simulink model "complex_dbe_core"  (Simulink 7.1)
settings: Solver=ode45  StartTime=0.0  StopTime=1000  RelTol=1e-3
libraries: xbsIndex_r4 x308, cfa_library x64, casper_library_misc x6, simulink x2
(part 3 of 6)

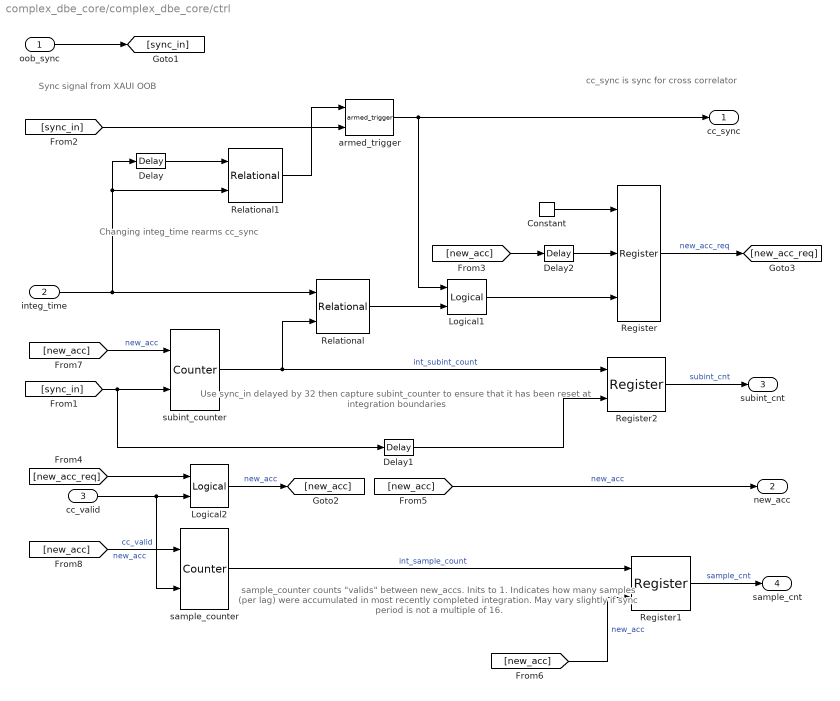
== system complex_dbe_core/complex_dbe_core/ctrl ==
  note: Sync signal from XAUI OOB
  note: cc_sync is sync for
      | cross correlator
  note: Changing integ_time
      | rearms cc_sync
  note: Use sync_in delayed by 32 then capture subint_counter to
      | ensure that it has been reset at integration boundaries
  note: sample_counter counts "valids" between new_accs.  Inits to 1.
      | Indicates how many samples (per lag) were accumulated
      | in most recently completed integration.  May vary slightly if
      | sync period is not a multiple of 16.
  oob_sync : Inport
  integ_time : Inport  Port=2
  cc_valid : Inport  Port=3
  Constant : xbsIndex_r4/Constant  arith_type=Boolean  const=1  n_bits=16  bin_pt=14  explicit_period=on  period=1  equ=P=C  opselect=C  inp2=PCIN>>17  opr=+  inp1=P  carry=CIN  dbl_ovrd=off  block_type=constant
  Delay : xbsIndex_r4/Delay  en=off  latency=1  dbl_ovrd=off  reg_retiming=off  block_type=delay
  Delay1 : xbsIndex_r4/Delay  en=off  latency=32  dbl_ovrd=off  reg_retiming=off  block_type=delay
  Delay2 : xbsIndex_r4/Delay  en=off  latency=2  dbl_ovrd=off  reg_retiming=off  block_type=delay
  Logical1 : xbsIndex_r4/Logical  logical_function=OR  inputs=2  en=off  latency=0  precision=Full  arith_type=Unsigned  n_bits=16  bin_pt=0  align_bp=on  dbl_ovrd=off  block_type=logical
  Logical2 : xbsIndex_r4/Logical  logical_function=AND  inputs=2  en=off  latency=0  precision=Full  arith_type=Unsigned  n_bits=16  bin_pt=0  align_bp=on  dbl_ovrd=off  block_type=logical
  Register : xbsIndex_r4/Register  init=0  rst=on  en=on  dbl_ovrd=off  block_type=register
  Register1 : xbsIndex_r4/Register  init=0  rst=off  en=on  dbl_ovrd=off  block_type=register
  Register2 : xbsIndex_r4/Register  init=0  rst=off  en=on  dbl_ovrd=off  block_type=register
  Relational : xbsIndex_r4/Relational  mode=a=b  en=off  latency=1  dbl_ovrd=off  block_type=relational
      settings: block_version=10.1.3
  Relational1 : xbsIndex_r4/Relational  mode=a=b  en=off  latency=1  dbl_ovrd=off  block_type=relational
      settings: block_version=10.1.3
  armed_trigger : casper_library_misc/armed_trigger  SystemSampleTime=-1  hidden=0
  sample_counter : xbsIndex_r4/Counter  cnt_type=Free Running  cnt_to=Inf  operation=Up  start_count=1  cnt_by_val=1  arith_type=Unsigned  n_bits=32  bin_pt=0  load_pin=off  rst=on  en=on  explicit_period=on  period=1  dbl_ovrd=off  use_behavioral_HDL=off  use_rpm=off  implementation=Fabric  block_type=counter
  subint_counter : xbsIndex_r4/Counter  cnt_type=Free Running  cnt_to=Inf  operation=Up  start_count=0  cnt_by_val=1  arith_type=Unsigned  n_bits=32  bin_pt=0  load_pin=off  rst=on  en=on  explicit_period=on  period=1  dbl_ovrd=off  use_behavioral_HDL=off  use_rpm=off  implementation=Fabric  block_type=counter
  cc_sync : Outport
  new_acc : Outport  Port=2
  subint_cnt : Outport  Port=3
  sample_cnt : Outport  Port=4
  wires:
  armed_trigger/1 -> cc_sync/1, Logical1/1
  oob_sync/1 -> [sync_in]
  [new_acc] -> subint_counter/1  "new_acc"
  [sync_in] -> subint_counter/2, Delay1/1
  integ_time/1 -> Delay/1, Relational1/2, Relational/1
  Relational/1 -> Logical1/2
  Logical1/1 -> Register/3
  Delay/1 -> Relational1/1
  subint_counter/1 -> Relational/2, Register2/1  "int_subint_count"
  Relational1/1 -> armed_trigger/1
  [sync_in] -> armed_trigger/2
  Register/1 -> [new_acc_req]  "new_acc_req"
  [new_acc] -> Delay2/1
  Constant/1 -> Register/1
  Delay2/1 -> Register/2
  Delay1/1 -> Register2/2
  Register2/1 -> subint_cnt/1  "subint_cnt"
  [new_acc_req] -> Logical2/1
  cc_valid/1 -> Logical2/2, sample_counter/2  "cc_valid"
  Logical2/1 -> [new_acc]  "new_acc"
  [new_acc] -> new_acc/1  "new_acc"
  [new_acc] -> sample_counter/1  "new_acc"
  sample_counter/1 -> Register1/1  "int_sample_count"
  [new_acc] -> Register1/2  "new_acc"
  Register1/1 -> sample_cnt/1  "sample_cnt"

== system complex_dbe_core/complex_dbe_core/edge_detect ==
  in : Inport  OutDataType=sfix(16)  OutScaling=2^0
  Delay : xbsIndex_r4/Delay  en=off  latency=1  dbl_ovrd=off  reg_retiming=off  block_type=delay
      settings: xl_area=[0, 0, 0, 0, 0, 0, 0]
  Inverter : xbsIndex_r4/Inverter  en=off  latency=0  dbl_ovrd=off  block_type=inv
      settings: xl_area=[0, 0, 0, 0, 0, 0, 0]
  edge_op : xbsIndex_r4/Logical  logical_function=AND  inputs=2  en=off  latency=0  precision=Full  arith_type=Unsigned  n_bits=8  bin_pt=2  align_bp=on  dbl_ovrd=off  block_type=logical
      settings: xl_area=[0, 0, 0, 0, 0, 0, 0]
  out : Outport  OutDataType=sfix(16)  OutScaling=2^0
  wires:
  Inverter/1 -> edge_op/1
  edge_op/1 -> out/1
  in/1 -> Inverter/1, Delay/1
  Delay/1 -> edge_op/2

== system complex_dbe_core/complex_dbe_core/edge_detect1 ==
  in : Inport  OutDataType=sfix(16)  OutScaling=2^0
  Delay : xbsIndex_r4/Delay  en=off  latency=1  dbl_ovrd=off  reg_retiming=off  block_type=delay
      settings: xl_area=[0, 0, 0, 0, 0, 0, 0]
  Inverter : xbsIndex_r4/Inverter  en=off  latency=0  dbl_ovrd=off  block_type=inv
      settings: xl_area=[0, 0, 0, 0, 0, 0, 0]
  edge_op : xbsIndex_r4/Logical  logical_function=AND  inputs=2  en=off  latency=0  precision=Full  arith_type=Unsigned  n_bits=8  bin_pt=2  align_bp=on  dbl_ovrd=off  block_type=logical
      settings: xl_area=[0, 0, 0, 0, 0, 0, 0]
  out : Outport  OutDataType=sfix(16)  OutScaling=2^0
  wires:
  Inverter/1 -> edge_op/1
  edge_op/1 -> out/1
  in/1 -> Inverter/1, Delay/1
  Delay/1 -> edge_op/2

== system complex_dbe_core/complex_dbe_core/usb_imag_bram_vacc ==
  new_acc : Inport
  din : Inport  Port=2
  Delay1 : xbsIndex_r4/Delay  en=off  latency=1  dbl_ovrd=off  reg_retiming=off  block_type=delay
  Delay2 : xbsIndex_r4/Delay  en=off  latency=1  dbl_ovrd=off  reg_retiming=off  block_type=delay
  Delay5 : xbsIndex_r4/Delay  en=off  latency=2  dbl_ovrd=off  reg_retiming=off  block_type=delay
      settings: block_version=11.4
  Delay6 : xbsIndex_r4/Delay  en=off  latency=2  dbl_ovrd=off  reg_retiming=off  block_type=delay
      settings: block_version=11.4
  Reinterpret : xbsIndex_r4/Reinterpret  force_arith_type=off  arith_type=Unsigned  force_bin_pt=on  bin_pt=4  block_type=reinterpret
      settings: infoedit="Changes signal type without altering the binary representation.   You can changed the signal between signed and unsigned, and relocate the binary point.<P><P>Hardware notes: In hardware this block costs nothing.<P><P>Example:  Suppose the input is 6 bits wide, signed, with 2 fractional bits, and the output is forced to unsigned with 0 fractional bits.  Then an input of -2.0 (1110.00 in binary 2's complement) becomes an output of 56 (111000 in binary)."  block_version=10.1.3
  addr_bram_vacc : Subsystem  AncestorBlock=casper_library_accumulators/addr_bram_vacc  mask(simple_bram_vacc){vec_len=16, arith_type=Signed, n_bits=36, bin_pt=0}
      mask prompts: vec_len "Vector length:"; arith_type "Output type:"; n_bits "Bit width (output):"; bin_pt "Binary point (output):"
      mask help: This simple vector accumulator is based on a shift register. It outputs its previous accumulated vector after a new_acc pulse is received.
      mask init:
      | simple_bram_vacc_init(gcb, ...
      |     'vec_len', vec_len, ...
      |     'arith_type', arith_type, ...
      |     'n_bits', n_bits, ...
      |     'bin_pt', bin_pt);
      mask StyleString: edit,popup(Signed|Unsigned),edit,edit
  convert : Subsystem  AncestorBlock=casper_library_misc/convert  mask(convert){bin_pt_in=4, n_bits_out=32, bin_pt_out=0, quantization=Round  (unbiased: Even Values), overflow=Wrap, latency=1}
      mask prompts: bin_pt_in "Binary Point In"; n_bits_out "Bit Width Out"; bin_pt_out "Binary Point Out"
      mask help:
      | Convert input value to the specified bit width and precision.
      |
      | Does not support upscaling number of fractional bits (eg 8_5 to 8_4 is ok, but not 8_4 to 8_5).
      mask init:
      | convert_init(gcb, ...
      |     'bin_pt_in',bin_pt_in, ...
      |     'n_bits_out',n_bits_out,...
      |     'bin_pt_out',bin_pt_out, ...
      |     'quantization',quantization,...
      |     'overflow',overflow,...
      |     'latency',latency);
      settings: AttributesFormatString=|
      | N_4 ==> 32_0
      | round even, wrap
      | latency = 1
      mask Help:
      | <pre>
      | Description::
      | 
      | Outputs converted version of the input.
      | 
      | Mask Parameters::
      | 
      | Binary Point In (bin_pt_in): Specifies the binary point location in the input.
      | 
      | Bit Width Out (n_bits_out): Specifies the width of the output.
      | 
      | Binary Point Out (bin_pt_out): Specifies the binary point location in the output.
      | 
      | Quantization (quantization): Specifies quantization handling.
      | 
      | Overflow (overflow): Specifies overflow handling.
      | 
      | Latency (latency): Specifies the latency of the underlying adder block, which is the overall
      | latency of this block as well.
      | </pre>
      mask StyleString: edit,edit,edit,popup(Truncate|Round  (unbiased: +/- Inf)|Round  (unbiased: Even Values)|Round  (unbiased: Zero)|Round  (unbiased: Odd Values)|Round  (biased: Up)|Round  (biased: Down)),popup(Wrap|Saturate|Error),edit
  addr : Outport
  dout : Outport  Port=2
  we : Outport  Port=3
  wires:
  Delay5/1 -> addr_bram_vacc/1(new_acc)  "bv_new_acc"
  Delay6/1 -> addr_bram_vacc/2(din)  "bv_din"
  new_acc/1 -> Delay5/1
  addr_bram_vacc/2(dout) -> Reinterpret/1
  din/1 -> Delay6/1
  addr_bram_vacc/3(we) -> Delay2/1
  addr_bram_vacc/1(addr) -> Delay1/1
  Reinterpret/1 -> convert/1(in)
  convert/1(out) -> dout/1
  Delay1/1 -> addr/1
  Delay2/1 -> we/1

== system complex_dbe_core/complex_dbe_core/usb_real_bram_vacc ==
  new_acc : Inport
  din : Inport  Port=2
  Delay1 : xbsIndex_r4/Delay  en=off  latency=1  dbl_ovrd=off  reg_retiming=off  block_type=delay
  Delay2 : xbsIndex_r4/Delay  en=off  latency=1  dbl_ovrd=off  reg_retiming=off  block_type=delay
  Delay5 : xbsIndex_r4/Delay  en=off  latency=2  dbl_ovrd=off  reg_retiming=off  block_type=delay
      settings: block_version=11.4
  Delay6 : xbsIndex_r4/Delay  en=off  latency=2  dbl_ovrd=off  reg_retiming=off  block_type=delay
      settings: block_version=11.4
  Reinterpret : xbsIndex_r4/Reinterpret  force_arith_type=off  arith_type=Unsigned  force_bin_pt=on  bin_pt=4  block_type=reinterpret
      settings: infoedit="Changes signal type without altering the binary representation.   You can changed the signal between signed and unsigned, and relocate the binary point.<P><P>Hardware notes: In hardware this block costs nothing.<P><P>Example:  Suppose the input is 6 bits wide, signed, with 2 fractional bits, and the output is forced to unsigned with 0 fractional bits.  Then an input of -2.0 (1110.00 in binary 2's complement) becomes an output of 56 (111000 in binary)."  block_version=10.1.3
  addr_bram_vacc : Subsystem  AncestorBlock=casper_library_accumulators/addr_bram_vacc  mask(simple_bram_vacc){vec_len=16, arith_type=Signed, n_bits=36, bin_pt=0}
      mask prompts: vec_len "Vector length:"; arith_type "Output type:"; n_bits "Bit width (output):"; bin_pt "Binary point (output):"
      mask help: This simple vector accumulator is based on a shift register. It outputs its previous accumulated vector after a new_acc pulse is received.
      mask init:
      | simple_bram_vacc_init(gcb, ...
      |     'vec_len', vec_len, ...
      |     'arith_type', arith_type, ...
      |     'n_bits', n_bits, ...
      |     'bin_pt', bin_pt);
      mask StyleString: edit,popup(Signed|Unsigned),edit,edit
  convert : Subsystem  AncestorBlock=casper_library_misc/convert  mask(convert){bin_pt_in=4, n_bits_out=32, bin_pt_out=0, quantization=Round  (unbiased: Even Values), overflow=Wrap, latency=1}
      mask prompts: bin_pt_in "Binary Point In"; n_bits_out "Bit Width Out"; bin_pt_out "Binary Point Out"
      mask help:
      | Convert input value to the specified bit width and precision.
      |
      | Does not support upscaling number of fractional bits (eg 8_5 to 8_4 is ok, but not 8_4 to 8_5).
      mask init: same as complex_dbe_core/complex_dbe_core/usb_imag_bram_vacc/convert
      settings: AttributesFormatString=|
      | N_4 ==> 32_0
      | round even, wrap
      | latency = 1
      mask Help:
      | <pre>
      | Description::
      | 
      | Outputs converted version of the input.
      | 
      | Mask Parameters::
      | 
      | Binary Point In (bin_pt_in): Specifies the binary point location in the input.
      | 
      | Bit Width Out (n_bits_out): Specifies the width of the output.
      | 
      | Binary Point Out (bin_pt_out): Specifies the binary point location in the output.
      | 
      | Quantization (quantization): Specifies quantization handling.
      | 
      | Overflow (overflow): Specifies overflow handling.
      | 
      | Latency (latency): Specifies the latency of the underlying adder block, which is the overall
      | latency of this block as well.
      | </pre>
      mask StyleString: edit,edit,edit,popup(Truncate|Round  (unbiased: +/- Inf)|Round  (unbiased: Even Values)|Round  (unbiased: Zero)|Round  (unbiased: Odd Values)|Round  (biased: Up)|Round  (biased: Down)),popup(Wrap|Saturate|Error),edit
  addr : Outport
  dout : Outport  Port=2
  we : Outport  Port=3
  wires:
  Delay5/1 -> addr_bram_vacc/1(new_acc)  "bv_new_acc"
  Delay6/1 -> addr_bram_vacc/2(din)  "bv_din"
  new_acc/1 -> Delay5/1
  addr_bram_vacc/2(dout) -> Reinterpret/1
  din/1 -> Delay6/1
  addr_bram_vacc/3(we) -> Delay2/1
  addr_bram_vacc/1(addr) -> Delay1/1
  Reinterpret/1 -> convert/1(in)
  convert/1(out) -> dout/1
  Delay1/1 -> addr/1
  Delay2/1 -> we/1

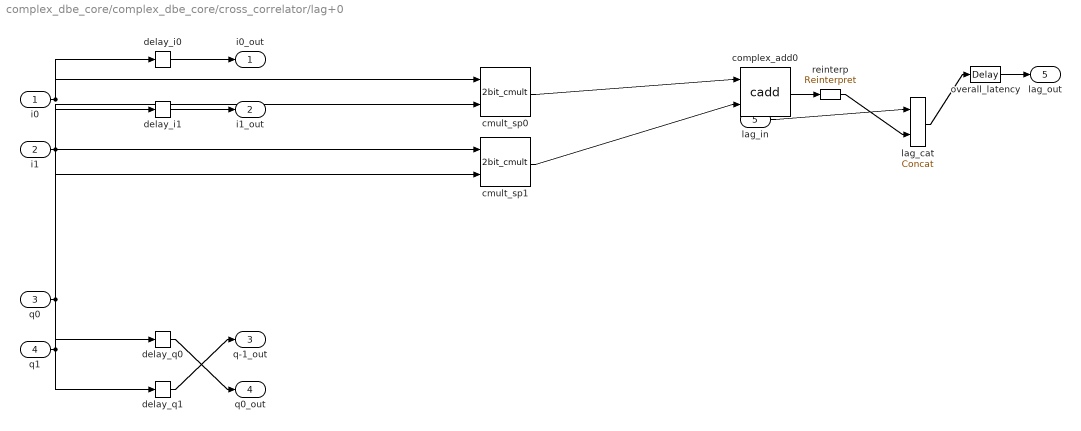
== system complex_dbe_core/complex_dbe_core/cross_correlator/lag+0 ==
  i0 : Inport
  i1 : Inport  Port=2
  q0 : Inport  Port=3
  q1 : Inport  Port=4
  lag_in : Inport  Port=5
  cmult_sp0 : cfa_library/2bit_cmult  SystemSampleTime=-1  add_delay=2
  cmult_sp1 : cfa_library/2bit_cmult  SystemSampleTime=-1  add_delay=2
  complex_add0 : cfa_library/cadd  SystemSampleTime=-1  input_bit_width=6  input_bin_pt=0  add_delay=2
  delay_i0 : xbsIndex_r4/Delay  en=off  latency=2  dbl_ovrd=off  reg_retiming=off  block_type=delay
      settings: block_version=11.4
  delay_i1 : xbsIndex_r4/Delay  en=off  latency=2  dbl_ovrd=off  reg_retiming=off  block_type=delay
      settings: block_version=11.4
  delay_q0 : xbsIndex_r4/Delay  en=off  latency=1  dbl_ovrd=off  reg_retiming=off  block_type=delay
      settings: block_version=11.4
  delay_q1 : xbsIndex_r4/Delay  en=off  latency=2  dbl_ovrd=off  reg_retiming=off  block_type=delay
      settings: block_version=11.4
  lag_cat : xbsIndex_r4/Concat  num_inputs=2  dbl_ovrd=off  block_type=concat
  overall_latency : xbsIndex_r4/Delay  en=off  latency=2  dbl_ovrd=off  reg_retiming=on  block_type=delay
  reinterp : xbsIndex_r4/Reinterpret  force_arith_type=on  arith_type=Unsigned  force_bin_pt=on  bin_pt=0  block_type=reinterpret
      settings: infoedit="Changes signal type without altering the binary representation.   You can changed the signal between signed and unsigned, and relocate the binary point.<br><br>Hardware notes: In hardware this block costs nothing.<br><br>Example:  Suppose the input is 6 bits wide, signed, with 2 fractional bits, and the output is forced to unsigned with 0 fractional bits.  Then an input of -2.0 (1110.00 in binary 2's complement) becomes an output of 56 (111000 in binary)."
  i0_out : Outport
  i1_out : Outport  Port=2
  q-1_out : Outport  Port=3
  q0_out : Outport  Port=4
  lag_out : Outport  Port=5
  wires:
  i0/1 -> cmult_sp0/1, delay_i0/1
  q0/1 -> cmult_sp0/2, delay_q0/1
  i1/1 -> cmult_sp1/1, delay_i1/1
  q1/1 -> cmult_sp1/2, delay_q1/1
  cmult_sp0/1 -> complex_add0/1
  cmult_sp1/1 -> complex_add0/2
  delay_i0/1 -> i0_out/1
  delay_q0/1 -> q0_out/1
  delay_i1/1 -> i1_out/1
  delay_q1/1 -> q-1_out/1
  lag_in/1 -> lag_cat/1
  complex_add0/1 -> reinterp/1
  reinterp/1 -> lag_cat/2
  lag_cat/1 -> overall_latency/1
  overall_latency/1 -> lag_out/1

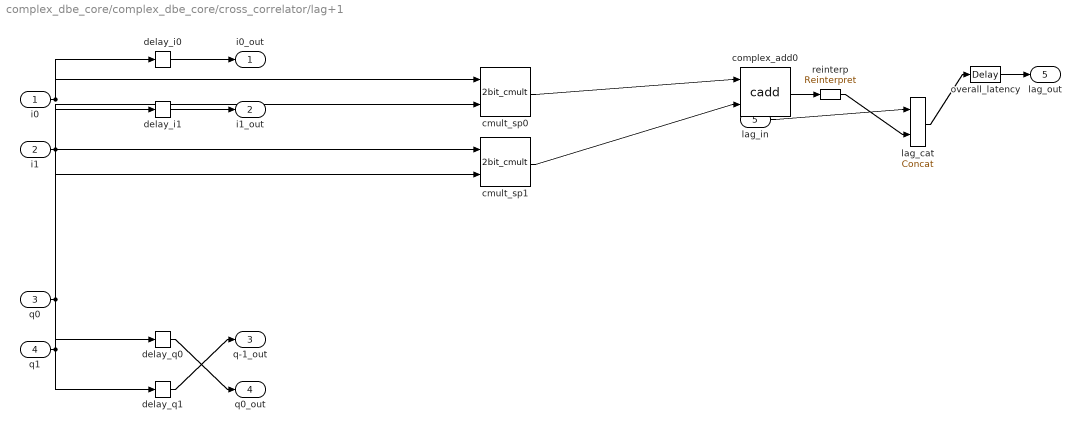
== system complex_dbe_core/complex_dbe_core/cross_correlator/lag+1 ==
  i0 : Inport
  i1 : Inport  Port=2
  q0 : Inport  Port=3
  q1 : Inport  Port=4
  lag_in : Inport  Port=5
  cmult_sp0 : cfa_library/2bit_cmult  SystemSampleTime=-1  add_delay=2
  cmult_sp1 : cfa_library/2bit_cmult  SystemSampleTime=-1  add_delay=2
  complex_add0 : cfa_library/cadd  SystemSampleTime=-1  input_bit_width=6  input_bin_pt=0  add_delay=2
  delay_i0 : xbsIndex_r4/Delay  en=off  latency=2  dbl_ovrd=off  reg_retiming=off  block_type=delay
      settings: block_version=11.4
  delay_i1 : xbsIndex_r4/Delay  en=off  latency=2  dbl_ovrd=off  reg_retiming=off  block_type=delay
      settings: block_version=11.4
  delay_q0 : xbsIndex_r4/Delay  en=off  latency=1  dbl_ovrd=off  reg_retiming=off  block_type=delay
      settings: block_version=11.4
  delay_q1 : xbsIndex_r4/Delay  en=off  latency=2  dbl_ovrd=off  reg_retiming=off  block_type=delay
      settings: block_version=11.4
  lag_cat : xbsIndex_r4/Concat  num_inputs=2  dbl_ovrd=off  block_type=concat
  overall_latency : xbsIndex_r4/Delay  en=off  latency=2  dbl_ovrd=off  reg_retiming=on  block_type=delay
  reinterp : xbsIndex_r4/Reinterpret  force_arith_type=on  arith_type=Unsigned  force_bin_pt=on  bin_pt=0  block_type=reinterpret
      settings: infoedit="Changes signal type without altering the binary representation.   You can changed the signal between signed and unsigned, and relocate the binary point.<br><br>Hardware notes: In hardware this block costs nothing.<br><br>Example:  Suppose the input is 6 bits wide, signed, with 2 fractional bits, and the output is forced to unsigned with 0 fractional bits.  Then an input of -2.0 (1110.00 in binary 2's complement) becomes an output of 56 (111000 in binary)."
  i0_out : Outport
  i1_out : Outport  Port=2
  q-1_out : Outport  Port=3
  q0_out : Outport  Port=4
  lag_out : Outport  Port=5
  wires:
  i0/1 -> cmult_sp0/1, delay_i0/1
  q0/1 -> cmult_sp0/2, delay_q0/1
  i1/1 -> cmult_sp1/1, delay_i1/1
  q1/1 -> cmult_sp1/2, delay_q1/1
  cmult_sp0/1 -> complex_add0/1
  cmult_sp1/1 -> complex_add0/2
  delay_i0/1 -> i0_out/1
  delay_q0/1 -> q0_out/1
  delay_i1/1 -> i1_out/1
  delay_q1/1 -> q-1_out/1
  lag_in/1 -> lag_cat/1
  complex_add0/1 -> reinterp/1
  reinterp/1 -> lag_cat/2
  lag_cat/1 -> overall_latency/1
  overall_latency/1 -> lag_out/1

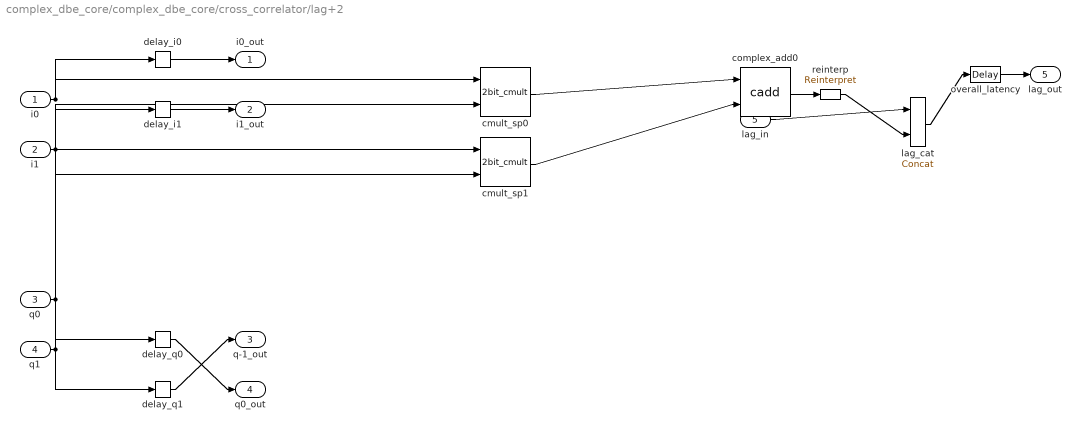
== system complex_dbe_core/complex_dbe_core/cross_correlator/lag+2 ==
  i0 : Inport
  i1 : Inport  Port=2
  q0 : Inport  Port=3
  q1 : Inport  Port=4
  lag_in : Inport  Port=5
  cmult_sp0 : cfa_library/2bit_cmult  SystemSampleTime=-1  add_delay=2
  cmult_sp1 : cfa_library/2bit_cmult  SystemSampleTime=-1  add_delay=2
  complex_add0 : cfa_library/cadd  SystemSampleTime=-1  input_bit_width=6  input_bin_pt=0  add_delay=2
  delay_i0 : xbsIndex_r4/Delay  en=off  latency=2  dbl_ovrd=off  reg_retiming=off  block_type=delay
      settings: block_version=11.4
  delay_i1 : xbsIndex_r4/Delay  en=off  latency=2  dbl_ovrd=off  reg_retiming=off  block_type=delay
      settings: block_version=11.4
  delay_q0 : xbsIndex_r4/Delay  en=off  latency=1  dbl_ovrd=off  reg_retiming=off  block_type=delay
      settings: block_version=11.4
  delay_q1 : xbsIndex_r4/Delay  en=off  latency=2  dbl_ovrd=off  reg_retiming=off  block_type=delay
      settings: block_version=11.4
  lag_cat : xbsIndex_r4/Concat  num_inputs=2  dbl_ovrd=off  block_type=concat
  overall_latency : xbsIndex_r4/Delay  en=off  latency=2  dbl_ovrd=off  reg_retiming=on  block_type=delay
  reinterp : xbsIndex_r4/Reinterpret  force_arith_type=on  arith_type=Unsigned  force_bin_pt=on  bin_pt=0  block_type=reinterpret
      settings: infoedit="Changes signal type without altering the binary representation.   You can changed the signal between signed and unsigned, and relocate the binary point.<br><br>Hardware notes: In hardware this block costs nothing.<br><br>Example:  Suppose the input is 6 bits wide, signed, with 2 fractional bits, and the output is forced to unsigned with 0 fractional bits.  Then an input of -2.0 (1110.00 in binary 2's complement) becomes an output of 56 (111000 in binary)."
  i0_out : Outport
  i1_out : Outport  Port=2
  q-1_out : Outport  Port=3
  q0_out : Outport  Port=4
  lag_out : Outport  Port=5
  wires:
  i0/1 -> cmult_sp0/1, delay_i0/1
  q0/1 -> cmult_sp0/2, delay_q0/1
  i1/1 -> cmult_sp1/1, delay_i1/1
  q1/1 -> cmult_sp1/2, delay_q1/1
  cmult_sp0/1 -> complex_add0/1
  cmult_sp1/1 -> complex_add0/2
  delay_i0/1 -> i0_out/1
  delay_q0/1 -> q0_out/1
  delay_i1/1 -> i1_out/1
  delay_q1/1 -> q-1_out/1
  lag_in/1 -> lag_cat/1
  complex_add0/1 -> reinterp/1
  reinterp/1 -> lag_cat/2
  lag_cat/1 -> overall_latency/1
  overall_latency/1 -> lag_out/1

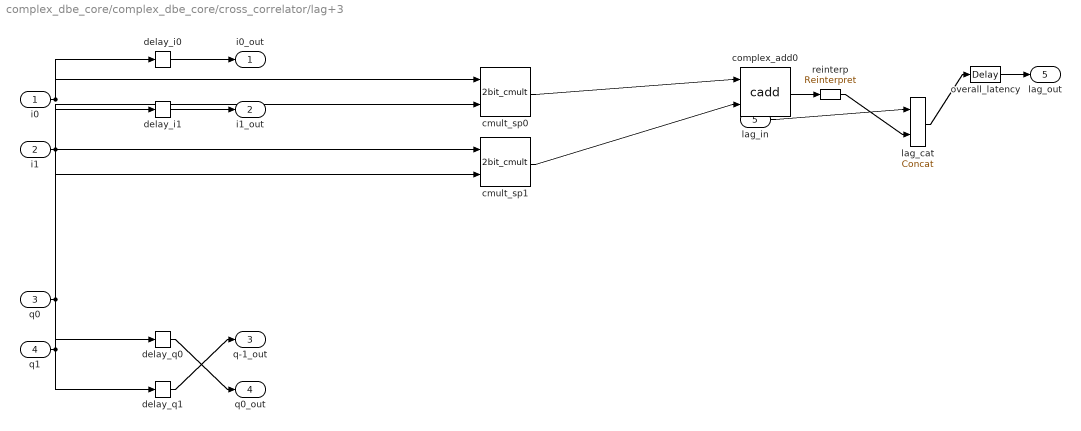
== system complex_dbe_core/complex_dbe_core/cross_correlator/lag+3 ==
  i0 : Inport
  i1 : Inport  Port=2
  q0 : Inport  Port=3
  q1 : Inport  Port=4
  lag_in : Inport  Port=5
  cmult_sp0 : cfa_library/2bit_cmult  SystemSampleTime=-1  add_delay=2
  cmult_sp1 : cfa_library/2bit_cmult  SystemSampleTime=-1  add_delay=2
  complex_add0 : cfa_library/cadd  SystemSampleTime=-1  input_bit_width=6  input_bin_pt=0  add_delay=2
  delay_i0 : xbsIndex_r4/Delay  en=off  latency=2  dbl_ovrd=off  reg_retiming=off  block_type=delay
      settings: block_version=11.4
  delay_i1 : xbsIndex_r4/Delay  en=off  latency=2  dbl_ovrd=off  reg_retiming=off  block_type=delay
      settings: block_version=11.4
  delay_q0 : xbsIndex_r4/Delay  en=off  latency=1  dbl_ovrd=off  reg_retiming=off  block_type=delay
      settings: block_version=11.4
  delay_q1 : xbsIndex_r4/Delay  en=off  latency=2  dbl_ovrd=off  reg_retiming=off  block_type=delay
      settings: block_version=11.4
  lag_cat : xbsIndex_r4/Concat  num_inputs=2  dbl_ovrd=off  block_type=concat
  overall_latency : xbsIndex_r4/Delay  en=off  latency=2  dbl_ovrd=off  reg_retiming=on  block_type=delay
  reinterp : xbsIndex_r4/Reinterpret  force_arith_type=on  arith_type=Unsigned  force_bin_pt=on  bin_pt=0  block_type=reinterpret
      settings: infoedit="Changes signal type without altering the binary representation.   You can changed the signal between signed and unsigned, and relocate the binary point.<br><br>Hardware notes: In hardware this block costs nothing.<br><br>Example:  Suppose the input is 6 bits wide, signed, with 2 fractional bits, and the output is forced to unsigned with 0 fractional bits.  Then an input of -2.0 (1110.00 in binary 2's complement) becomes an output of 56 (111000 in binary)."
  i0_out : Outport
  i1_out : Outport  Port=2
  q-1_out : Outport  Port=3
  q0_out : Outport  Port=4
  lag_out : Outport  Port=5
  wires:
  i0/1 -> cmult_sp0/1, delay_i0/1
  q0/1 -> cmult_sp0/2, delay_q0/1
  i1/1 -> cmult_sp1/1, delay_i1/1
  q1/1 -> cmult_sp1/2, delay_q1/1
  cmult_sp0/1 -> complex_add0/1
  cmult_sp1/1 -> complex_add0/2
  delay_i0/1 -> i0_out/1
  delay_q0/1 -> q0_out/1
  delay_i1/1 -> i1_out/1
  delay_q1/1 -> q-1_out/1
  lag_in/1 -> lag_cat/1
  complex_add0/1 -> reinterp/1
  reinterp/1 -> lag_cat/2
  lag_cat/1 -> overall_latency/1
  overall_latency/1 -> lag_out/1

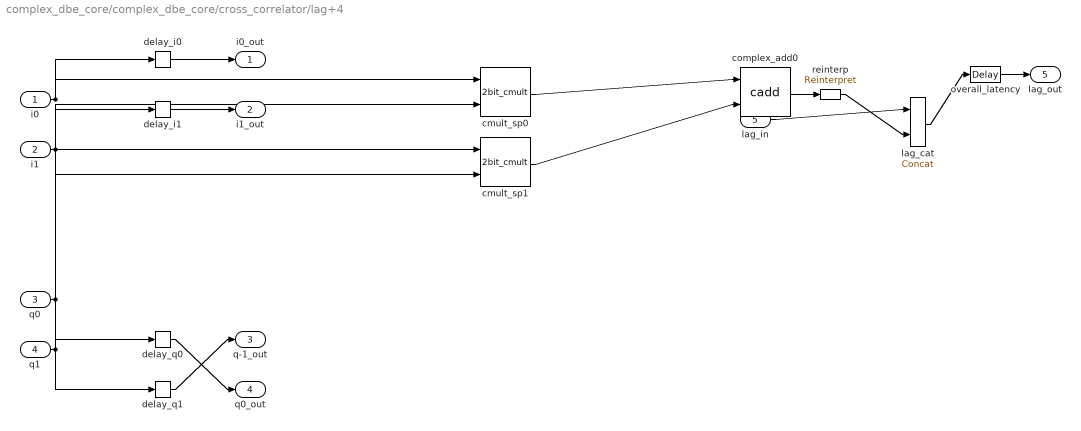
== system complex_dbe_core/complex_dbe_core/cross_correlator/lag+4 ==
  i0 : Inport
  i1 : Inport  Port=2
  q0 : Inport  Port=3
  q1 : Inport  Port=4
  lag_in : Inport  Port=5
  cmult_sp0 : cfa_library/2bit_cmult  SystemSampleTime=-1  add_delay=2
  cmult_sp1 : cfa_library/2bit_cmult  SystemSampleTime=-1  add_delay=2
  complex_add0 : cfa_library/cadd  SystemSampleTime=-1  input_bit_width=6  input_bin_pt=0  add_delay=2
  delay_i0 : xbsIndex_r4/Delay  en=off  latency=2  dbl_ovrd=off  reg_retiming=off  block_type=delay
      settings: block_version=11.4
  delay_i1 : xbsIndex_r4/Delay  en=off  latency=2  dbl_ovrd=off  reg_retiming=off  block_type=delay
      settings: block_version=11.4
  delay_q0 : xbsIndex_r4/Delay  en=off  latency=1  dbl_ovrd=off  reg_retiming=off  block_type=delay
      settings: block_version=11.4
  delay_q1 : xbsIndex_r4/Delay  en=off  latency=2  dbl_ovrd=off  reg_retiming=off  block_type=delay
      settings: block_version=11.4
  lag_cat : xbsIndex_r4/Concat  num_inputs=2  dbl_ovrd=off  block_type=concat
  overall_latency : xbsIndex_r4/Delay  en=off  latency=2  dbl_ovrd=off  reg_retiming=on  block_type=delay
  reinterp : xbsIndex_r4/Reinterpret  force_arith_type=on  arith_type=Unsigned  force_bin_pt=on  bin_pt=0  block_type=reinterpret
      settings: infoedit="Changes signal type without altering the binary representation.   You can changed the signal between signed and unsigned, and relocate the binary point.<br><br>Hardware notes: In hardware this block costs nothing.<br><br>Example:  Suppose the input is 6 bits wide, signed, with 2 fractional bits, and the output is forced to unsigned with 0 fractional bits.  Then an input of -2.0 (1110.00 in binary 2's complement) becomes an output of 56 (111000 in binary)."
  i0_out : Outport
  i1_out : Outport  Port=2
  q-1_out : Outport  Port=3
  q0_out : Outport  Port=4
  lag_out : Outport  Port=5
  wires:
  i0/1 -> cmult_sp0/1, delay_i0/1
  q0/1 -> cmult_sp0/2, delay_q0/1
  i1/1 -> cmult_sp1/1, delay_i1/1
  q1/1 -> cmult_sp1/2, delay_q1/1
  cmult_sp0/1 -> complex_add0/1
  cmult_sp1/1 -> complex_add0/2
  delay_i0/1 -> i0_out/1
  delay_q0/1 -> q0_out/1
  delay_i1/1 -> i1_out/1
  delay_q1/1 -> q-1_out/1
  lag_in/1 -> lag_cat/1
  complex_add0/1 -> reinterp/1
  reinterp/1 -> lag_cat/2
  lag_cat/1 -> overall_latency/1
  overall_latency/1 -> lag_out/1

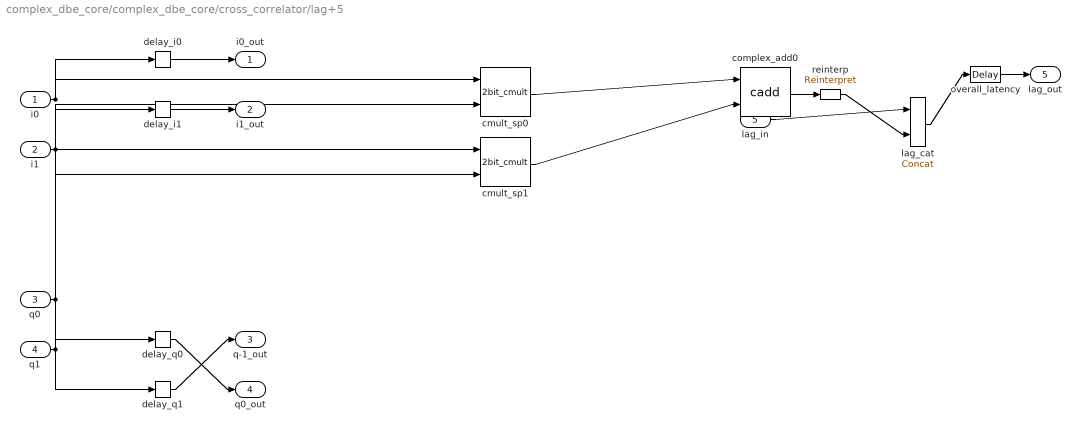
== system complex_dbe_core/complex_dbe_core/cross_correlator/lag+5 ==
  i0 : Inport
  i1 : Inport  Port=2
  q0 : Inport  Port=3
  q1 : Inport  Port=4
  lag_in : Inport  Port=5
  cmult_sp0 : cfa_library/2bit_cmult  SystemSampleTime=-1  add_delay=2
  cmult_sp1 : cfa_library/2bit_cmult  SystemSampleTime=-1  add_delay=2
  complex_add0 : cfa_library/cadd  SystemSampleTime=-1  input_bit_width=6  input_bin_pt=0  add_delay=2
  delay_i0 : xbsIndex_r4/Delay  en=off  latency=2  dbl_ovrd=off  reg_retiming=off  block_type=delay
      settings: block_version=11.4
  delay_i1 : xbsIndex_r4/Delay  en=off  latency=2  dbl_ovrd=off  reg_retiming=off  block_type=delay
      settings: block_version=11.4
  delay_q0 : xbsIndex_r4/Delay  en=off  latency=1  dbl_ovrd=off  reg_retiming=off  block_type=delay
      settings: block_version=11.4
  delay_q1 : xbsIndex_r4/Delay  en=off  latency=2  dbl_ovrd=off  reg_retiming=off  block_type=delay
      settings: block_version=11.4
  lag_cat : xbsIndex_r4/Concat  num_inputs=2  dbl_ovrd=off  block_type=concat
  overall_latency : xbsIndex_r4/Delay  en=off  latency=2  dbl_ovrd=off  reg_retiming=on  block_type=delay
  reinterp : xbsIndex_r4/Reinterpret  force_arith_type=on  arith_type=Unsigned  force_bin_pt=on  bin_pt=0  block_type=reinterpret
      settings: infoedit="Changes signal type without altering the binary representation.   You can changed the signal between signed and unsigned, and relocate the binary point.<br><br>Hardware notes: In hardware this block costs nothing.<br><br>Example:  Suppose the input is 6 bits wide, signed, with 2 fractional bits, and the output is forced to unsigned with 0 fractional bits.  Then an input of -2.0 (1110.00 in binary 2's complement) becomes an output of 56 (111000 in binary)."
  i0_out : Outport
  i1_out : Outport  Port=2
  q-1_out : Outport  Port=3
  q0_out : Outport  Port=4
  lag_out : Outport  Port=5
  wires:
  i0/1 -> cmult_sp0/1, delay_i0/1
  q0/1 -> cmult_sp0/2, delay_q0/1
  i1/1 -> cmult_sp1/1, delay_i1/1
  q1/1 -> cmult_sp1/2, delay_q1/1
  cmult_sp0/1 -> complex_add0/1
  cmult_sp1/1 -> complex_add0/2
  delay_i0/1 -> i0_out/1
  delay_q0/1 -> q0_out/1
  delay_i1/1 -> i1_out/1
  delay_q1/1 -> q-1_out/1
  lag_in/1 -> lag_cat/1
  complex_add0/1 -> reinterp/1
  reinterp/1 -> lag_cat/2
  lag_cat/1 -> overall_latency/1
  overall_latency/1 -> lag_out/1

== system complex_dbe_core/complex_dbe_core/cross_correlator/lag+6 ==
  i0 : Inport
  i1 : Inport  Port=2
  q0 : Inport  Port=3
  q1 : Inport  Port=4
  lag_in : Inport  Port=5
  cmult_sp0 : cfa_library/2bit_cmult  SystemSampleTime=-1  add_delay=2
  cmult_sp1 : cfa_library/2bit_cmult  SystemSampleTime=-1  add_delay=2
  complex_add0 : cfa_library/cadd  SystemSampleTime=-1  input_bit_width=6  input_bin_pt=0  add_delay=2
  delay_i0 : xbsIndex_r4/Delay  en=off  latency=2  dbl_ovrd=off  reg_retiming=off  block_type=delay
      settings: block_version=11.4
  delay_i1 : xbsIndex_r4/Delay  en=off  latency=2  dbl_ovrd=off  reg_retiming=off  block_type=delay
      settings: block_version=11.4
  delay_q0 : xbsIndex_r4/Delay  en=off  latency=1  dbl_ovrd=off  reg_retiming=off  block_type=delay
      settings: block_version=11.4
  delay_q1 : xbsIndex_r4/Delay  en=off  latency=2  dbl_ovrd=off  reg_retiming=off  block_type=delay
      settings: block_version=11.4
  lag_cat : xbsIndex_r4/Concat  num_inputs=2  dbl_ovrd=off  block_type=concat
  overall_latency : xbsIndex_r4/Delay  en=off  latency=2  dbl_ovrd=off  reg_retiming=on  block_type=delay
  reinterp : xbsIndex_r4/Reinterpret  force_arith_type=on  arith_type=Unsigned  force_bin_pt=on  bin_pt=0  block_type=reinterpret
      settings: infoedit="Changes signal type without altering the binary representation.   You can changed the signal between signed and unsigned, and relocate the binary point.<br><br>Hardware notes: In hardware this block costs nothing.<br><br>Example:  Suppose the input is 6 bits wide, signed, with 2 fractional bits, and the output is forced to unsigned with 0 fractional bits.  Then an input of -2.0 (1110.00 in binary 2's complement) becomes an output of 56 (111000 in binary)."
  i0_out : Outport
  i1_out : Outport  Port=2
  q-1_out : Outport  Port=3
  q0_out : Outport  Port=4
  lag_out : Outport  Port=5
  wires:
  i0/1 -> cmult_sp0/1, delay_i0/1
  q0/1 -> cmult_sp0/2, delay_q0/1
  i1/1 -> cmult_sp1/1, delay_i1/1
  q1/1 -> cmult_sp1/2, delay_q1/1
  cmult_sp0/1 -> complex_add0/1
  cmult_sp1/1 -> complex_add0/2
  delay_i0/1 -> i0_out/1
  delay_q0/1 -> q0_out/1
  delay_i1/1 -> i1_out/1
  delay_q1/1 -> q-1_out/1
  lag_in/1 -> lag_cat/1
  complex_add0/1 -> reinterp/1
  reinterp/1 -> lag_cat/2
  lag_cat/1 -> overall_latency/1
  overall_latency/1 -> lag_out/1

== system complex_dbe_core/complex_dbe_core/cross_correlator/lag+7 ==
  i0 : Inport
  i1 : Inport  Port=2
  q0 : Inport  Port=3
  q1 : Inport  Port=4
  lag_in : Inport  Port=5
  cmult_sp0 : cfa_library/2bit_cmult  SystemSampleTime=-1  add_delay=2
  cmult_sp1 : cfa_library/2bit_cmult  SystemSampleTime=-1  add_delay=2
  complex_add0 : cfa_library/cadd  SystemSampleTime=-1  input_bit_width=6  input_bin_pt=0  add_delay=2
  delay_i0 : xbsIndex_r4/Delay  en=off  latency=2  dbl_ovrd=off  reg_retiming=off  block_type=delay
      settings: block_version=11.4
  delay_i1 : xbsIndex_r4/Delay  en=off  latency=2  dbl_ovrd=off  reg_retiming=off  block_type=delay
      settings: block_version=11.4
  delay_q0 : xbsIndex_r4/Delay  en=off  latency=1  dbl_ovrd=off  reg_retiming=off  block_type=delay
      settings: block_version=11.4
  delay_q1 : xbsIndex_r4/Delay  en=off  latency=2  dbl_ovrd=off  reg_retiming=off  block_type=delay
      settings: block_version=11.4
  lag_cat : xbsIndex_r4/Concat  num_inputs=2  dbl_ovrd=off  block_type=concat
  overall_latency : xbsIndex_r4/Delay  en=off  latency=2  dbl_ovrd=off  reg_retiming=on  block_type=delay
  reinterp : xbsIndex_r4/Reinterpret  force_arith_type=on  arith_type=Unsigned  force_bin_pt=on  bin_pt=0  block_type=reinterpret
      settings: infoedit="Changes signal type without altering the binary representation.   You can changed the signal between signed and unsigned, and relocate the binary point.<br><br>Hardware notes: In hardware this block costs nothing.<br><br>Example:  Suppose the input is 6 bits wide, signed, with 2 fractional bits, and the output is forced to unsigned with 0 fractional bits.  Then an input of -2.0 (1110.00 in binary 2's complement) becomes an output of 56 (111000 in binary)."
  i0_out : Outport
  i1_out : Outport  Port=2
  q-1_out : Outport  Port=3
  q0_out : Outport  Port=4
  lag_out : Outport  Port=5
  wires:
  i0/1 -> cmult_sp0/1, delay_i0/1
  q0/1 -> cmult_sp0/2, delay_q0/1
  i1/1 -> cmult_sp1/1, delay_i1/1
  q1/1 -> cmult_sp1/2, delay_q1/1
  cmult_sp0/1 -> complex_add0/1
  cmult_sp1/1 -> complex_add0/2
  delay_i0/1 -> i0_out/1
  delay_q0/1 -> q0_out/1
  delay_i1/1 -> i1_out/1
  delay_q1/1 -> q-1_out/1
  lag_in/1 -> lag_cat/1
  complex_add0/1 -> reinterp/1
  reinterp/1 -> lag_cat/2
  lag_cat/1 -> overall_latency/1
  overall_latency/1 -> lag_out/1

== system complex_dbe_core/complex_dbe_core/cross_correlator/lag-1 ==
  i0 : Inport
  i1 : Inport  Port=2
  q0 : Inport  Port=3
  q1 : Inport  Port=4
  lag_in : Inport  Port=5
  cmult_sp0 : cfa_library/2bit_cmult  SystemSampleTime=-1  add_delay=2
  cmult_sp1 : cfa_library/2bit_cmult  SystemSampleTime=-1  add_delay=2
  complex_add0 : cfa_library/cadd  SystemSampleTime=-1  input_bit_width=6  input_bin_pt=0  add_delay=2
  delay_i0 : xbsIndex_r4/Delay  en=off  latency=1  dbl_ovrd=off  reg_retiming=off  block_type=delay
      settings: block_version=11.4
  delay_i1 : xbsIndex_r4/Delay  en=off  latency=2  dbl_ovrd=off  reg_retiming=off  block_type=delay
      settings: block_version=11.4
  delay_q0 : xbsIndex_r4/Delay  en=off  latency=1  dbl_ovrd=off  reg_retiming=off  block_type=delay
      settings: block_version=11.4
  delay_q1 : xbsIndex_r4/Delay  en=off  latency=1  dbl_ovrd=off  reg_retiming=off  block_type=delay
      settings: block_version=11.4
  lag_cat : xbsIndex_r4/Concat  num_inputs=2  dbl_ovrd=off  block_type=concat
  overall_latency : xbsIndex_r4/Delay  en=off  latency=1  dbl_ovrd=off  reg_retiming=on  block_type=delay
  reinterp : xbsIndex_r4/Reinterpret  force_arith_type=on  arith_type=Unsigned  force_bin_pt=on  bin_pt=0  block_type=reinterpret
      settings: infoedit="Changes signal type without altering the binary representation.   You can changed the signal between signed and unsigned, and relocate the binary point.<br><br>Hardware notes: In hardware this block costs nothing.<br><br>Example:  Suppose the input is 6 bits wide, signed, with 2 fractional bits, and the output is forced to unsigned with 0 fractional bits.  Then an input of -2.0 (1110.00 in binary 2's complement) becomes an output of 56 (111000 in binary)."
  i-1_out : Outport
  i0_out : Outport  Port=2
  q0_out : Outport  Port=3
  q1_out : Outport  Port=4
  lag_out : Outport  Port=5
  wires:
  i0/1 -> cmult_sp0/1, delay_i0/1
  q0/1 -> cmult_sp0/2, delay_q0/1
  i1/1 -> cmult_sp1/1, delay_i1/1
  q1/1 -> cmult_sp1/2, delay_q1/1
  cmult_sp0/1 -> complex_add0/1
  cmult_sp1/1 -> complex_add0/2
  delay_i0/1 -> i0_out/1
  delay_q0/1 -> q0_out/1
  delay_i1/1 -> i-1_out/1
  delay_q1/1 -> q1_out/1
  lag_in/1 -> lag_cat/1
  complex_add0/1 -> reinterp/1
  reinterp/1 -> lag_cat/2
  lag_cat/1 -> overall_latency/1
  overall_latency/1 -> lag_out/1

== system complex_dbe_core/complex_dbe_core/cross_correlator/lag-2 ==
  i0 : Inport
  i1 : Inport  Port=2
  q0 : Inport  Port=3
  q1 : Inport  Port=4
  lag_in : Inport  Port=5
  cmult_sp0 : cfa_library/2bit_cmult  SystemSampleTime=-1  add_delay=2
  cmult_sp1 : cfa_library/2bit_cmult  SystemSampleTime=-1  add_delay=2
  complex_add0 : cfa_library/cadd  SystemSampleTime=-1  input_bit_width=6  input_bin_pt=0  add_delay=2
  delay_i0 : xbsIndex_r4/Delay  en=off  latency=1  dbl_ovrd=off  reg_retiming=off  block_type=delay
      settings: block_version=11.4
  delay_i1 : xbsIndex_r4/Delay  en=off  latency=2  dbl_ovrd=off  reg_retiming=off  block_type=delay
      settings: block_version=11.4
  delay_q0 : xbsIndex_r4/Delay  en=off  latency=1  dbl_ovrd=off  reg_retiming=off  block_type=delay
      settings: block_version=11.4
  delay_q1 : xbsIndex_r4/Delay  en=off  latency=1  dbl_ovrd=off  reg_retiming=off  block_type=delay
      settings: block_version=11.4
  lag_cat : xbsIndex_r4/Concat  num_inputs=2  dbl_ovrd=off  block_type=concat
  overall_latency : xbsIndex_r4/Delay  en=off  latency=1  dbl_ovrd=off  reg_retiming=on  block_type=delay
  reinterp : xbsIndex_r4/Reinterpret  force_arith_type=on  arith_type=Unsigned  force_bin_pt=on  bin_pt=0  block_type=reinterpret
      settings: infoedit="Changes signal type without altering the binary representation.   You can changed the signal between signed and unsigned, and relocate the binary point.<br><br>Hardware notes: In hardware this block costs nothing.<br><br>Example:  Suppose the input is 6 bits wide, signed, with 2 fractional bits, and the output is forced to unsigned with 0 fractional bits.  Then an input of -2.0 (1110.00 in binary 2's complement) becomes an output of 56 (111000 in binary)."
  i-1_out : Outport
  i0_out : Outport  Port=2
  q0_out : Outport  Port=3
  q1_out : Outport  Port=4
  lag_out : Outport  Port=5
  wires:
  i0/1 -> cmult_sp0/1, delay_i0/1
  q0/1 -> cmult_sp0/2, delay_q0/1
  i1/1 -> cmult_sp1/1, delay_i1/1
  q1/1 -> cmult_sp1/2, delay_q1/1
  cmult_sp0/1 -> complex_add0/1
  cmult_sp1/1 -> complex_add0/2
  delay_i0/1 -> i0_out/1
  delay_q0/1 -> q0_out/1
  delay_i1/1 -> i-1_out/1
  delay_q1/1 -> q1_out/1
  lag_in/1 -> lag_cat/1
  complex_add0/1 -> reinterp/1
  reinterp/1 -> lag_cat/2
  lag_cat/1 -> overall_latency/1
  overall_latency/1 -> lag_out/1

== system complex_dbe_core/complex_dbe_core/cross_correlator/lag-3 ==
  i0 : Inport
  i1 : Inport  Port=2
  q0 : Inport  Port=3
  q1 : Inport  Port=4
  lag_in : Inport  Port=5
  cmult_sp0 : cfa_library/2bit_cmult  SystemSampleTime=-1  add_delay=2
  cmult_sp1 : cfa_library/2bit_cmult  SystemSampleTime=-1  add_delay=2
  complex_add0 : cfa_library/cadd  SystemSampleTime=-1  input_bit_width=6  input_bin_pt=0  add_delay=2
  delay_i0 : xbsIndex_r4/Delay  en=off  latency=1  dbl_ovrd=off  reg_retiming=off  block_type=delay
      settings: block_version=11.4
  delay_i1 : xbsIndex_r4/Delay  en=off  latency=2  dbl_ovrd=off  reg_retiming=off  block_type=delay
      settings: block_version=11.4
  delay_q0 : xbsIndex_r4/Delay  en=off  latency=1  dbl_ovrd=off  reg_retiming=off  block_type=delay
      settings: block_version=11.4
  delay_q1 : xbsIndex_r4/Delay  en=off  latency=1  dbl_ovrd=off  reg_retiming=off  block_type=delay
      settings: block_version=11.4
  lag_cat : xbsIndex_r4/Concat  num_inputs=2  dbl_ovrd=off  block_type=concat
  overall_latency : xbsIndex_r4/Delay  en=off  latency=1  dbl_ovrd=off  reg_retiming=on  block_type=delay
  reinterp : xbsIndex_r4/Reinterpret  force_arith_type=on  arith_type=Unsigned  force_bin_pt=on  bin_pt=0  block_type=reinterpret
      settings: infoedit="Changes signal type without altering the binary representation.   You can changed the signal between signed and unsigned, and relocate the binary point.<br><br>Hardware notes: In hardware this block costs nothing.<br><br>Example:  Suppose the input is 6 bits wide, signed, with 2 fractional bits, and the output is forced to unsigned with 0 fractional bits.  Then an input of -2.0 (1110.00 in binary 2's complement) becomes an output of 56 (111000 in binary)."
  i-1_out : Outport
  i0_out : Outport  Port=2
  q0_out : Outport  Port=3
  q1_out : Outport  Port=4
  lag_out : Outport  Port=5
  wires:
  i0/1 -> cmult_sp0/1, delay_i0/1
  q0/1 -> cmult_sp0/2, delay_q0/1
  i1/1 -> cmult_sp1/1, delay_i1/1
  q1/1 -> cmult_sp1/2, delay_q1/1
  cmult_sp0/1 -> complex_add0/1
  cmult_sp1/1 -> complex_add0/2
  delay_i0/1 -> i0_out/1
  delay_q0/1 -> q0_out/1
  delay_i1/1 -> i-1_out/1
  delay_q1/1 -> q1_out/1
  lag_in/1 -> lag_cat/1
  complex_add0/1 -> reinterp/1
  reinterp/1 -> lag_cat/2
  lag_cat/1 -> overall_latency/1
  overall_latency/1 -> lag_out/1

== system complex_dbe_core/complex_dbe_core/cross_correlator/lag-4 ==
  i0 : Inport
  i1 : Inport  Port=2
  q0 : Inport  Port=3
  q1 : Inport  Port=4
  lag_in : Inport  Port=5
  cmult_sp0 : cfa_library/2bit_cmult  SystemSampleTime=-1  add_delay=2
  cmult_sp1 : cfa_library/2bit_cmult  SystemSampleTime=-1  add_delay=2
  complex_add0 : cfa_library/cadd  SystemSampleTime=-1  input_bit_width=6  input_bin_pt=0  add_delay=2
  delay_i0 : xbsIndex_r4/Delay  en=off  latency=1  dbl_ovrd=off  reg_retiming=off  block_type=delay
      settings: block_version=11.4
  delay_i1 : xbsIndex_r4/Delay  en=off  latency=2  dbl_ovrd=off  reg_retiming=off  block_type=delay
      settings: block_version=11.4
  delay_q0 : xbsIndex_r4/Delay  en=off  latency=1  dbl_ovrd=off  reg_retiming=off  block_type=delay
      settings: block_version=11.4
  delay_q1 : xbsIndex_r4/Delay  en=off  latency=1  dbl_ovrd=off  reg_retiming=off  block_type=delay
      settings: block_version=11.4
  lag_cat : xbsIndex_r4/Concat  num_inputs=2  dbl_ovrd=off  block_type=concat
  overall_latency : xbsIndex_r4/Delay  en=off  latency=1  dbl_ovrd=off  reg_retiming=on  block_type=delay
  reinterp : xbsIndex_r4/Reinterpret  force_arith_type=on  arith_type=Unsigned  force_bin_pt=on  bin_pt=0  block_type=reinterpret
      settings: infoedit="Changes signal type without altering the binary representation.   You can changed the signal between signed and unsigned, and relocate the binary point.<br><br>Hardware notes: In hardware this block costs nothing.<br><br>Example:  Suppose the input is 6 bits wide, signed, with 2 fractional bits, and the output is forced to unsigned with 0 fractional bits.  Then an input of -2.0 (1110.00 in binary 2's complement) becomes an output of 56 (111000 in binary)."
  i-1_out : Outport
  i0_out : Outport  Port=2
  q0_out : Outport  Port=3
  q1_out : Outport  Port=4
  lag_out : Outport  Port=5
  wires:
  i0/1 -> cmult_sp0/1, delay_i0/1
  q0/1 -> cmult_sp0/2, delay_q0/1
  i1/1 -> cmult_sp1/1, delay_i1/1
  q1/1 -> cmult_sp1/2, delay_q1/1
  cmult_sp0/1 -> complex_add0/1
  cmult_sp1/1 -> complex_add0/2
  delay_i0/1 -> i0_out/1
  delay_q0/1 -> q0_out/1
  delay_i1/1 -> i-1_out/1
  delay_q1/1 -> q1_out/1
  lag_in/1 -> lag_cat/1
  complex_add0/1 -> reinterp/1
  reinterp/1 -> lag_cat/2
  lag_cat/1 -> overall_latency/1
  overall_latency/1 -> lag_out/1

== system complex_dbe_core/complex_dbe_core/cross_correlator/lag-5 ==
  i0 : Inport
  i1 : Inport  Port=2
  q0 : Inport  Port=3
  q1 : Inport  Port=4
  lag_in : Inport  Port=5
  cmult_sp0 : cfa_library/2bit_cmult  SystemSampleTime=-1  add_delay=2
  cmult_sp1 : cfa_library/2bit_cmult  SystemSampleTime=-1  add_delay=2
  complex_add0 : cfa_library/cadd  SystemSampleTime=-1  input_bit_width=6  input_bin_pt=0  add_delay=2
  delay_i0 : xbsIndex_r4/Delay  en=off  latency=1  dbl_ovrd=off  reg_retiming=off  block_type=delay
      settings: block_version=11.4
  delay_i1 : xbsIndex_r4/Delay  en=off  latency=2  dbl_ovrd=off  reg_retiming=off  block_type=delay
      settings: block_version=11.4
  delay_q0 : xbsIndex_r4/Delay  en=off  latency=1  dbl_ovrd=off  reg_retiming=off  block_type=delay
      settings: block_version=11.4
  delay_q1 : xbsIndex_r4/Delay  en=off  latency=1  dbl_ovrd=off  reg_retiming=off  block_type=delay
      settings: block_version=11.4
  lag_cat : xbsIndex_r4/Concat  num_inputs=2  dbl_ovrd=off  block_type=concat
  overall_latency : xbsIndex_r4/Delay  en=off  latency=1  dbl_ovrd=off  reg_retiming=on  block_type=delay
  reinterp : xbsIndex_r4/Reinterpret  force_arith_type=on  arith_type=Unsigned  force_bin_pt=on  bin_pt=0  block_type=reinterpret
      settings: infoedit="Changes signal type without altering the binary representation.   You can changed the signal between signed and unsigned, and relocate the binary point.<br><br>Hardware notes: In hardware this block costs nothing.<br><br>Example:  Suppose the input is 6 bits wide, signed, with 2 fractional bits, and the output is forced to unsigned with 0 fractional bits.  Then an input of -2.0 (1110.00 in binary 2's complement) becomes an output of 56 (111000 in binary)."
  i-1_out : Outport
  i0_out : Outport  Port=2
  q0_out : Outport  Port=3
  q1_out : Outport  Port=4
  lag_out : Outport  Port=5
  wires:
  i0/1 -> cmult_sp0/1, delay_i0/1
  q0/1 -> cmult_sp0/2, delay_q0/1
  i1/1 -> cmult_sp1/1, delay_i1/1
  q1/1 -> cmult_sp1/2, delay_q1/1
  cmult_sp0/1 -> complex_add0/1
  cmult_sp1/1 -> complex_add0/2
  delay_i0/1 -> i0_out/1
  delay_q0/1 -> q0_out/1
  delay_i1/1 -> i-1_out/1
  delay_q1/1 -> q1_out/1
  lag_in/1 -> lag_cat/1
  complex_add0/1 -> reinterp/1
  reinterp/1 -> lag_cat/2
  lag_cat/1 -> overall_latency/1
  overall_latency/1 -> lag_out/1

== system complex_dbe_core/complex_dbe_core/cross_correlator/lag-6 ==
  i0 : Inport
  i1 : Inport  Port=2
  q0 : Inport  Port=3
  q1 : Inport  Port=4
  lag_in : Inport  Port=5
  cmult_sp0 : cfa_library/2bit_cmult  SystemSampleTime=-1  add_delay=2
  cmult_sp1 : cfa_library/2bit_cmult  SystemSampleTime=-1  add_delay=2
  complex_add0 : cfa_library/cadd  SystemSampleTime=-1  input_bit_width=6  input_bin_pt=0  add_delay=2
  delay_i0 : xbsIndex_r4/Delay  en=off  latency=1  dbl_ovrd=off  reg_retiming=off  block_type=delay
      settings: block_version=11.4
  delay_i1 : xbsIndex_r4/Delay  en=off  latency=2  dbl_ovrd=off  reg_retiming=off  block_type=delay
      settings: block_version=11.4
  delay_q0 : xbsIndex_r4/Delay  en=off  latency=1  dbl_ovrd=off  reg_retiming=off  block_type=delay
      settings: block_version=11.4
  delay_q1 : xbsIndex_r4/Delay  en=off  latency=1  dbl_ovrd=off  reg_retiming=off  block_type=delay
      settings: block_version=11.4
  lag_cat : xbsIndex_r4/Concat  num_inputs=2  dbl_ovrd=off  block_type=concat
  overall_latency : xbsIndex_r4/Delay  en=off  latency=1  dbl_ovrd=off  reg_retiming=on  block_type=delay
  reinterp : xbsIndex_r4/Reinterpret  force_arith_type=on  arith_type=Unsigned  force_bin_pt=on  bin_pt=0  block_type=reinterpret
      settings: infoedit="Changes signal type without altering the binary representation.   You can changed the signal between signed and unsigned, and relocate the binary point.<br><br>Hardware notes: In hardware this block costs nothing.<br><br>Example:  Suppose the input is 6 bits wide, signed, with 2 fractional bits, and the output is forced to unsigned with 0 fractional bits.  Then an input of -2.0 (1110.00 in binary 2's complement) becomes an output of 56 (111000 in binary)."
  i-1_out : Outport
  i0_out : Outport  Port=2
  q0_out : Outport  Port=3
  q1_out : Outport  Port=4
  lag_out : Outport  Port=5
  wires:
  i0/1 -> cmult_sp0/1, delay_i0/1
  q0/1 -> cmult_sp0/2, delay_q0/1
  i1/1 -> cmult_sp1/1, delay_i1/1
  q1/1 -> cmult_sp1/2, delay_q1/1
  cmult_sp0/1 -> complex_add0/1
  cmult_sp1/1 -> complex_add0/2
  delay_i0/1 -> i0_out/1
  delay_q0/1 -> q0_out/1
  delay_i1/1 -> i-1_out/1
  delay_q1/1 -> q1_out/1
  lag_in/1 -> lag_cat/1
  complex_add0/1 -> reinterp/1
  reinterp/1 -> lag_cat/2
  lag_cat/1 -> overall_latency/1
  overall_latency/1 -> lag_out/1

== system complex_dbe_core/complex_dbe_core/cross_correlator/lag-7 ==
  i0 : Inport
  i1 : Inport  Port=2
  q0 : Inport  Port=3
  q1 : Inport  Port=4
  lag_in : Inport  Port=5
  cmult_sp0 : cfa_library/2bit_cmult  SystemSampleTime=-1  add_delay=2
  cmult_sp1 : cfa_library/2bit_cmult  SystemSampleTime=-1  add_delay=2
  complex_add0 : cfa_library/cadd  SystemSampleTime=-1  input_bit_width=6  input_bin_pt=0  add_delay=2
  delay_i0 : xbsIndex_r4/Delay  en=off  latency=1  dbl_ovrd=off  reg_retiming=off  block_type=delay
      settings: block_version=11.4
  delay_i1 : xbsIndex_r4/Delay  en=off  latency=2  dbl_ovrd=off  reg_retiming=off  block_type=delay
      settings: block_version=11.4
  delay_q0 : xbsIndex_r4/Delay  en=off  latency=1  dbl_ovrd=off  reg_retiming=off  block_type=delay
      settings: block_version=11.4
  delay_q1 : xbsIndex_r4/Delay  en=off  latency=1  dbl_ovrd=off  reg_retiming=off  block_type=delay
      settings: block_version=11.4
  lag_cat : xbsIndex_r4/Concat  num_inputs=2  dbl_ovrd=off  block_type=concat
  overall_latency : xbsIndex_r4/Delay  en=off  latency=1  dbl_ovrd=off  reg_retiming=on  block_type=delay
  reinterp : xbsIndex_r4/Reinterpret  force_arith_type=on  arith_type=Unsigned  force_bin_pt=on  bin_pt=0  block_type=reinterpret
      settings: infoedit="Changes signal type without altering the binary representation.   You can changed the signal between signed and unsigned, and relocate the binary point.<br><br>Hardware notes: In hardware this block costs nothing.<br><br>Example:  Suppose the input is 6 bits wide, signed, with 2 fractional bits, and the output is forced to unsigned with 0 fractional bits.  Then an input of -2.0 (1110.00 in binary 2's complement) becomes an output of 56 (111000 in binary)."
  i-1_out : Outport
  i0_out : Outport  Port=2
  q0_out : Outport  Port=3
  q1_out : Outport  Port=4
  lag_out : Outport  Port=5
  wires:
  i0/1 -> cmult_sp0/1, delay_i0/1
  q0/1 -> cmult_sp0/2, delay_q0/1
  i1/1 -> cmult_sp1/1, delay_i1/1
  q1/1 -> cmult_sp1/2, delay_q1/1
  cmult_sp0/1 -> complex_add0/1
  cmult_sp1/1 -> complex_add0/2
  delay_i0/1 -> i0_out/1
  delay_q0/1 -> q0_out/1
  delay_i1/1 -> i-1_out/1
  delay_q1/1 -> q1_out/1
  lag_in/1 -> lag_cat/1
  complex_add0/1 -> reinterp/1
  reinterp/1 -> lag_cat/2
  lag_cat/1 -> overall_latency/1
  overall_latency/1 -> lag_out/1
